simulink model "EV_basic_8_1_triple"  (R2018b)
settings: Solver=VariableStepAuto  StartTime=0.0  StopTime=440  MaxStep=1e-2  MinStep=1e-5  RelTol=1e-2
values from neighbouring files (symbols this model uses):
  Av = 2.75    [InitiateModel.m]    (also in InitiateModel_layouts.m; nurburg_lap.mat)
  batt_max_v = cell_series*cell_max_v    [InitiateModel.m]    (also in nurburg_lap.mat = 613.2)
  Capacity = batt_cap*1e3*3600    (= 252000000)    [InitiateModel.m]    (also in InitiateModel_layouts.m = 252000; nurburg_lap.mat = 180000000)
  Cd = 0.26    [InitiateModel.m]    (also in InitiateModel_layouts.m; nurburg_lap.mat)
  Cr = 0.01    [InitiateModel.m]    (also in InitiateModel_layouts.m; nurburg_lap.mat)
  eta_DC = .985    (= 0.985)    [InitiateModel.m]    (also in InitiateModel_layouts.m; nurburg_lap.mat)
  eta_inv = .965    (= 0.965)    [InitiateModel.m]    (also in InitiateModel_layouts.m; nurburg_lap.mat)
  front_motor = 2    [InitiateModel.m]    (also in nurburg_lap.mat = 0)
  Fv_max = 2*Fv_max_electric    (= 22377.6223776)    [InitiateModel.m]    (also in InitiateModel_layouts.m = 16783.2167832; nurburg_lap.mat)
  Fz_tire = (Mv * weight_dist * 0.5)*9.81    [InitiateModel.m]    (also in nurburg_lap.mat = 5290.7414625)
  gratio = 7    [InitiateModel.m]    (also in InitiateModel_layouts.m = 5.3; nurburg_lap.mat = 5.5)
  grav = 9.81    [InitiateModel.m]    (also in InitiateModel_layouts.m; nurburg_lap.mat)
  inv_eff = 0.98    [InitiateModel.m]    (also in nurburg_lap.mat)
  Ke = 0.607    [InitiateModel.m]    (also in InitiateModel_layouts.m; nurburg_lap.mat)
  max_curr = cell_max_curr*cells_parallel    [InitiateModel.m]    (also in InitiateModel_layouts.m = 270; nurburg_lap.mat = 400)
  motoreff_T = linspace(0,300,101)    [InitiateModel.m]    (also in motoreff_w.mat = [0 4 8 12 16 20 24 28 32 36 40 44 ... (101 elements, 1x101)]; nurburg_lap.mat = [0 3 6 9 12 15 18 21 24 27 30 33 ... (101 elements, 1x101)])
  motoreff_w = [0 18 36 54 72 90 108 126 144 162 180 198 ... (101 elements, 1x101)]    [motoreff_w.mat]    (also in nurburg_lap.mat = [0 12 24 36 48 60 72 84 96 108 120 132 ... (101 elements, 1x)
  Mv = 1420    [InitiateModel.m]    (also in InitiateModel_layouts.m; nurburg_lap.mat)
  opt_slip = 0.18    [InitiateModel.m]    (also in nurburg_lap.mat)
  Pe_max = 160e3    (= 160000)    [InitiateModel.m]    (also in InitiateModel_layouts.m = 120000; nurburg_lap.mat)
  rear_motor = 2    [InitiateModel.m]    (also in nurburg_lap.mat)
  regen_eff = 0.8    [InitiateModel.m]    (also in nurburg_lap.mat)
  rho_air = 1.204    [InitiateModel.m]    (also in InitiateModel_layouts.m; nurburg_lap.mat)
  rw = 0.668/2    (= 0.334)    [InitiateModel.m]    (also in InitiateModel_layouts.m; nurburg_lap.mat)
  s_time = 0.01    [InitiateModel.m]    (also in InitiateModel_layouts.m; nurburg_lap.mat)
  SOC_0 = 80    [InitiateModel.m]    (also in InitiateModel_layouts.m; nurburg_lap.mat)
  Te_max = 2*Te_max_electric    (= 2442.52479547)    [InitiateModel.m]    (also in InitiateModel_layouts.m = 1831.8935966; nurburg_lap.mat)
  tstep = .01    (= 0.01)    [InitiateModel.m]    (also in InitiateModel_layouts.m; nurburg_lap.mat)
  Vbase = 14.30    (= 14.3)    [InitiateModel.m]    (also in InitiateModel_layouts.m; nurburg_lap.mat)
  Vbus_ref = 600    [InitiateModel.m]    (also in InitiateModel_layouts.m = 530; nurburg_lap.mat)
  W_d = 0.5    [InitiateModel.m]    (also in InitiateModel_layouts.m; nurburg_lap.mat)
undefined symbols (not defined in the file or in its folder): MException, throw
libraries: simulink x6, autolibshared x3, autolibdcdc x1
(part 4 of 4)

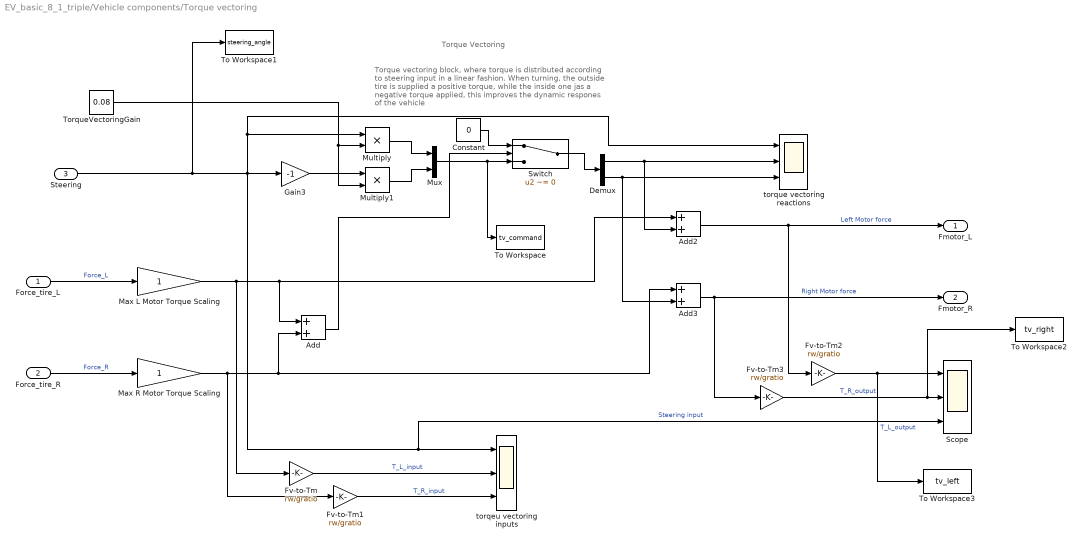
== system EV_basic_8_1_triple/Vehicle components/Torque vectoring ==
  note: Torque vectoring block, where torque is distributed according to steering input in a linear fashion.
      | When turning, the outside tire is supplied a positive torque, while the inside one jas a negative torque applied, this improves the dynamic respones of the vehicle
  note: Torque Vectoring
  Force_tire_L : Inport
  Force_tire_R : Inport  Port=2
  Steering : Inport  Port=3
  Add : Sum
  Add2 : Sum
  Add3 : Sum
  Constant : Constant  Value=0
  Demux : Demux  Outputs=2
  Fv-to-Tm{,1..3} (4 alike) : Gain  Gain=rw/gratio
  Gain3 : Gain  Gain=-1
  Max L Motor Torque Scaling : Gain
  Max R Motor Torque Scaling : Gain
  Multiply : Product  Inputs=**
  Multiply1 : Product  Inputs=**
  Mux : Mux  Inputs=2
  Scope : Scope  NumInputPorts=3
  Switch : Switch  Criteria=u2 ~= 0  Threshold=0.05  ZeroCross=off
  To Workspace : ToWorkspace  VariableName=tv_command  SaveFormat=Structure With Time  SampleTime=-1
  To Workspace1 : ToWorkspace  VariableName=steering_angle  SaveFormat=Structure With Time  SampleTime=-1
  To Workspace2 : ToWorkspace  VariableName=tv_right  SaveFormat=Structure With Time  SampleTime=s_time
  To Workspace3 : ToWorkspace  VariableName=tv_left  SaveFormat=Structure With Time  SampleTime=s_time
  TorqueVectoringGain : Constant  Value=0.08
  torqeu vectoring inputs : Scope  NumInputPorts=3
  torque vectoring reactions : Scope  NumInputPorts=3
  Fmotor_L : Outport
  Fmotor_R : Outport  Port=2
  wires:
  Demux/1 -> Add2/2, torque vectoring reactions/2
  Multiply/1 -> Mux/1
  TorqueVectoringGain/1 -> Multiply1/2, Multiply/2
  Multiply1/1 -> Mux/2
  Add/1 -> Switch/2
  Force_tire_L/1 -> Max L Motor Torque Scaling/1  "Force_L"
  Steering/1 -> To Workspace1/1, Multiply/1, torque vectoring reactions/1, Scope/3, torqeu vectoring inputs/1, Gain3/1  "Steering input"
  Add2/1 -> Fv-to-Tm2/1, Fmotor_L/1  "Left Motor force"
  Gain3/1 -> Multiply1/1
  Max L Motor Torque Scaling/1 -> Fv-to-Tm/1, Add/1, Add2/1
  Constant/1 -> Switch/1
  Switch/1 -> Demux/1
  Mux/1 -> To Workspace/1, Switch/3
  Add3/1 -> Fv-to-Tm3/1, Fmotor_R/1  "Right Motor force"
  Max R Motor Torque Scaling/1 -> Fv-to-Tm1/1, Add/2, Add3/1
  Force_tire_R/1 -> Max R Motor Torque Scaling/1  "Force_R"
  Fv-to-Tm1/1 -> torqeu vectoring inputs/3  "T_R_input"
  Fv-to-Tm/1 -> torqeu vectoring inputs/2  "T_L_input"
  Demux/2 -> torque vectoring reactions/3, Add3/2
  Fv-to-Tm2/1 -> To Workspace3/1, Scope/1  "T_L_output"
  Fv-to-Tm3/1 -> To Workspace2/1, Scope/2  "T_R_output"

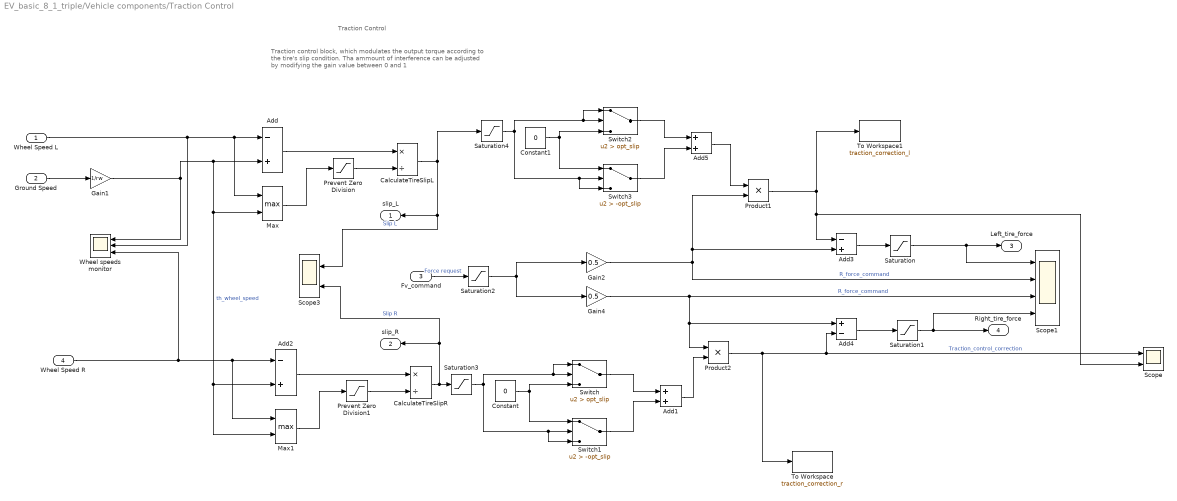
== system EV_basic_8_1_triple/Vehicle components/Traction Control ==
  note: Traction control block, which modulates the output torque according to the tire's slip condition. Tha ammount of interference can be adjusted by modifying the gain value between 0 and 1
  note: Traction Control
  Wheel Speed L : Inport
  Ground Speed : Inport  Port=2
  Fv_command : Inport  Port=3
  Wheel Speed R : Inport  Port=4
  Add : Sum  Inputs=-+
  Add1 : Sum
  Add2 : Sum  Inputs=-+
  Add3 : Sum  Inputs=-+
  Add4 : Sum  Inputs=+-
  Add5 : Sum
  CalculateTireSlipL : Product  Inputs=*/
  CalculateTireSlipR : Product  Inputs=*/
  Constant : Constant  Value=0
  Constant1 : Constant  Value=0
  Gain1 : Gain  Gain=1/rw
  Gain2 : Gain  Gain=0.5
  Gain4 : Gain  Gain=0.5
  Max : MinMax  Function=max  Inputs=2
  Max1 : MinMax  Function=max  Inputs=2
  Prevent Zero Division : Saturate  UpperLimit=1000  LowerLimit=0.0001
  Prevent Zero Division1 : Saturate  UpperLimit=1000  LowerLimit=0.0001
  Product1 : Product
  Product2 : Product
  Saturation : Saturate  UpperLimit=Te_max*(0.5*front_motor+0.5*rear_motor)*(gratio/rw)*0.5  LowerLimit=-Te_max*(0.5*front_motor+0.5*rear_motor)*(gratio/rw)*0.5
  Saturation1 : Saturate  UpperLimit=Te_max*(0.5*front_motor+0.5*rear_motor)*(gratio/rw)*0.5  LowerLimit=-Te_max*(0.5*front_motor+0.5*rear_motor)*(gratio/rw)*0.5
  Saturation2 : Saturate  UpperLimit=Te_max*(0.5*front_motor+0.5*rear_motor)*(gratio/rw)  LowerLimit=-Te_max*(0.5*front_motor+0.5*rear_motor)*(gratio/rw)
  Saturation3 : Saturate  UpperLimit=0.8  LowerLimit=-0.8
  Saturation4 : Saturate  UpperLimit=0.8  LowerLimit=-0.8
  Scope : Scope  NumInputPorts=2
  Scope1 : Scope  NumInputPorts=4
  Scope3 : Scope  NumInputPorts=2
  Switch : Switch  Criteria=u2 > Threshold  Threshold=opt_slip  ZeroCross=off
  Switch1 : Switch  Criteria=u2 > Threshold  Threshold=-opt_slip  ZeroCross=off
  Switch2 : Switch  Criteria=u2 > Threshold  Threshold=opt_slip  ZeroCross=off
  Switch3 : Switch  Criteria=u2 > Threshold  Threshold=-opt_slip  ZeroCross=off
  To Workspace : ToWorkspace  VariableName=traction_correction_r  SaveFormat=Structure With Time  SampleTime=s_time
  To Workspace1 : ToWorkspace  VariableName=traction_correction_l  SaveFormat=Structure With Time  SampleTime=s_time
  Wheel speeds monitor : Scope  NumInputPorts=3
  slip_L : Outport
  slip_R : Outport  Port=2
  Left_tire_force : Outport  Port=3
  Right_tire_force : Outport  Port=4
  wires:
  Prevent Zero Division/1 -> CalculateTireSlipL/2
  Max/1 -> Prevent Zero Division/1
  Wheel Speed L/1 -> Wheel speeds monitor/2, Max/1, Add/1
  Add/1 -> CalculateTireSlipL/1
  Wheel Speed R/1 -> Wheel speeds monitor/3, Max1/1, Add2/1
  Max1/1 -> Prevent Zero Division1/1
  Prevent Zero Division1/1 -> CalculateTireSlipR/2
  Ground Speed/1 -> Gain1/1
  Add2/1 -> CalculateTireSlipR/1
  Gain1/1 -> Max/2, Max1/2, Add2/2, Add/2, Wheel speeds monitor/1  "th_wheel_speed"
  Gain4/1 -> Product2/1, Add4/1, Scope1/3  "R_force_command"
  Fv_command/1 -> Saturation2/1  "Force request"
  Gain2/1 -> Add3/2, Product1/2, Scope1/2  "R_force_command"
  Saturation/1 -> Scope1/1, Left_tire_force/1
  Saturation1/1 -> Right_tire_force/1, Scope1/4
  Add3/1 -> Saturation/1
  Product2/1 -> To Workspace/1, Scope/1, Add4/2  "Traction_control_correction"
  CalculateTireSlipR/1 -> Scope3/2, slip_R/1, Saturation3/1  "Slip R"
  Add4/1 -> Saturation1/1
  Saturation2/1 -> Gain2/1, Gain4/1
  CalculateTireSlipL/1 -> Saturation4/1, Scope3/1, slip_L/1  "Slip L"
  Product1/1 -> To Workspace1/1, Scope/2, Add3/1
  Constant/1 -> Switch1/1, Switch/3
  Switch1/1 -> Add1/2
  Switch/1 -> Add1/1
  Add1/1 -> Product2/2
  Saturation3/1 -> Switch1/3, Switch1/2, Switch/1, Switch/2
  Switch2/1 -> Add5/1
  Saturation4/1 -> Switch3/3, Switch3/2, Switch2/1, Switch2/2
  Switch3/1 -> Add5/2
  Constant1/1 -> Switch3/1, Switch2/3
  Add5/1 -> Product1/1

== system EV_basic_8_1_triple/Vehicle components/Left Drive Inverter: Functional/Inverter Controller ==
  note: Inverter is kept in phase with rotor, and torque command is used
      | to directly set peak currents, which ultimately determine engine torque.
      | Because ideal sensing/control are assumed, no dynamics are considered
  note: Inverter Functional Controller
  Tactual : Inport
  thetar : Inport  Port=2
  Saturation : Saturate  UpperLimit=500  LowerLimit=-500
  Torque [Nm] to Inverter Peak Current [A] : Gain  Gain=1/Ke*2/3
  Ipk : Outport
  thetai : Outport  Port=2
  wires:
  thetar/1 -> thetai/1
  Torque [Nm] to Inverter Peak Current [A]/1 -> Saturation/1
  Tactual/1 -> Torque [Nm] to Inverter Peak Current [A]/1
  Saturation/1 -> Ipk/1

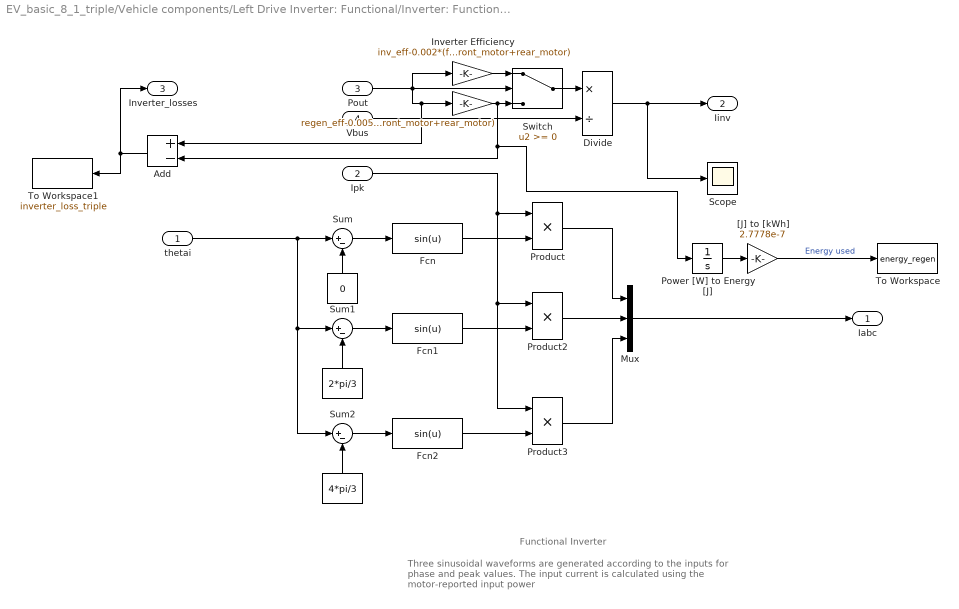
== system EV_basic_8_1_triple/Vehicle components/Left Drive Inverter: Functional/Inverter: Functional ==
  note: Three sinusoidal waveforms are generated according to the inputs
      | for phase and peak values.  The input current is calculated using
      | the motor-reported input power
  note: Functional Inverter
  thetai : Inport
  Ipk : Inport  Port=2
  Pout : Inport  Port=3
  Vbus : Inport  Port=4
  " " : Gain  Gain=regen_eff-0.005*(front_motor+rear_motor)
  " " : Constant  Value=0
  "   " : Constant  Value=2*pi/3
  "    " : Constant  Value=4*pi/3
  " Fcn" : Fcn  Expr=sin(u)
  Add : Sum  Inputs=+-
  Divide : Product  Inputs=*/
  Fcn1 : Fcn  Expr=sin(u)
  Fcn2 : Fcn  Expr=sin(u)
  Inverter Efficiency : Gain  Gain=inv_eff-0.002*(front_motor+rear_motor)
  Mux : Mux  Inputs=3
  Power [W] to Energy [J] : Integrator
  Product : Product  RndMeth=Zero
  Product2 : Product  RndMeth=Zero
  Product3 : Product  RndMeth=Zero
  Scope : Scope
  Sum : Sum  Inputs=|+-
  Sum1 : Sum  Inputs=|+-
  Sum2 : Sum  Inputs=|+-
  Switch : Switch
  To Workspace : ToWorkspace  VariableName=energy_regen  SaveFormat=Structure With Time  SampleTime=s_time
  To Workspace1 : ToWorkspace  VariableName=inverter_loss_triple  SaveFormat=Timeseries  SampleTime=-1
  "[J] to [kWh]" : Gain  Gain=2.7778e-7
  Iabc : Outport
  Iinv : Outport  Port=2
  Inverter_losses : Outport  Port=3
  wires:
  " Fcn"/1 -> Product/2
  Product/1 -> Mux/1
  Ipk/1 -> Product/1, Product2/1, Product3/1
  Sum/1 -> " Fcn"/1
  Fcn1/1 -> Product2/2
  Sum1/1 -> Fcn1/1
  Fcn2/1 -> Product3/2
  Sum2/1 -> Fcn2/1
  Product2/1 -> Mux/2
  Product3/1 -> Mux/3
  " "/1 -> Sum/2
  "   "/1 -> Sum1/2
  "    "/1 -> Sum2/2
  thetai/1 -> Sum/1, Sum1/1, Sum2/1
  Mux/1 -> Iabc/1
  Pout/1 -> Switch/2, Inverter Efficiency/1, Add/1, " "/1
  Vbus/1 -> Divide/2
  Divide/1 -> Scope/1, Iinv/1
  Switch/1 -> Divide/1
  Inverter Efficiency/1 -> Switch/1
  " "/1 -> Add/2, Power [W] to Energy [J]/1, Switch/3
  "[J] to [kWh]"/1 -> To Workspace/1  "Energy used"
  Power [W] to Energy [J]/1 -> "[J] to [kWh]"/1
  Add/1 -> To Workspace1/1, Inverter_losses/1

== system EV_basic_8_1_triple/Vehicle components/Left Drive Inverter: Functional/Motor Limits Model ==
  note: Electric Motor Limits Model
  note: Model enforces power and torque limits of engine
  wr : Inport
  Tmcommand : Inport  Port=2
  Engine Max Power : Saturate  UpperLimit=Pe_max*0.5*(0.5*front_motor+0.5*rear_motor)  LowerLimit=-Pe_max*0.5*(0.5*front_motor+0.5*rear_motor)
  Engine Max Torque : Saturate  UpperLimit=Te_max*1.3  LowerLimit=-Te_max*1.3
  Engine Max Torque1 : Saturate  UpperLimit=Te_max*0.5*(0.5*front_motor+0.5*rear_motor)  LowerLimit=-Te_max*0.5*(0.5*front_motor+0.5*rear_motor)
  Gearing Reduction : Gain  Gain=1/gratio
  Memory : Memory
  P=Tw : Product  RndMeth=Zero
  Scope : Scope  NumInputPorts=2
  Switch : Switch  Criteria=u2 ~= 0
  T=P/w : Product  Inputs=*/
  Torque or Power Limited Operation : simulink/Logic and Bit Operations/Compare To Constant  relop=<  const=Vbase  OutDataTypeStr=uint8  ZeroCross=off
  angular [rad/s]  to Linear [m/s] : Gain  Gain=rw
  Tactual : Outport
  wires:
  P=Tw/1 -> Engine Max Power/1  "Pm"
  Engine Max Power/1 -> T=P/w/1  "Pactual"
  Switch/1 -> Memory/1
  T=P/w/1 -> Engine Max Torque/1
  Torque or Power Limited Operation/1 -> Scope/1, Switch/2
  Memory/1 -> Tactual/1
  angular [rad/s]  to Linear [m/s]/1 -> Gearing Reduction/1
  wr/1 -> P=Tw/2, T=P/w/2, Scope/2, angular [rad/s]  to Linear [m/s]/1  "Rotor Angular Speed"
  Gearing Reduction/1 -> Torque or Power Limited Operation/1
  Engine Max Torque1/1 -> Switch/1
  Engine Max Torque/1 -> Switch/3
  Tmcommand/1 -> Engine Max Torque1/1, P=Tw/1

== system EV_basic_8_1_triple/Vehicle components/PMAC Motor Left: Functional/Ideal Motor Model ==
  note: Electric torque for PMAC is determined according to the three
      | current phases and their relative position to the rotor.
  note: PMAC Ideal Motor Electronic Torque Model
  Ia : Inport
  Ib : Inport  Port=2
  Ic : Inport  Port=3
  pihr : Inport  Port=4
  Add : Sum  Inputs=+++
  Angle between rotor and pole a : Fcn  Expr=sin(u)
  Angle between rotor and pole b : Fcn  Expr=sin(u-2*pi/3)
  Angle between rotor and pole c : Fcn  Expr=sin(u-4*pi/3)
  Product : Product  RndMeth=Zero
  Product1 : Product  RndMeth=Zero
  Product2 : Product  RndMeth=Zero
  Torque Constant : Gain  Gain=Ke
  Tm : Outport
  wires:
  pihr/1 -> Angle between rotor and pole a/1, Angle between rotor and pole b/1, Angle between rotor and pole c/1
  Angle between rotor and pole a/1 -> Product/2
  Ia/1 -> Product/1
  Ib/1 -> Product1/1
  Angle between rotor and pole b/1 -> Product1/2
  Ic/1 -> Product2/1
  Angle between rotor and pole c/1 -> Product2/2
  Add/1 -> Torque Constant/1
  Product/1 -> Add/1
  Product1/1 -> Add/2
  Product2/1 -> Add/3
  Torque Constant/1 -> Tm/1

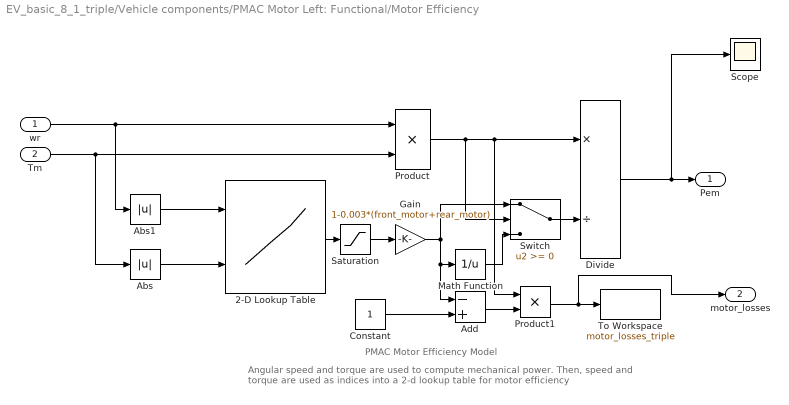
== system EV_basic_8_1_triple/Vehicle components/PMAC Motor Left: Functional/Motor Efficiency ==
  note: PMAC Motor Efficiency Model
  note: Angular speed and torque are used to compute mechanical power.  Then, speed
      | and torque are used as indices into a 2-d lookup table for motor efficiency
  wr : Inport
  Tm : Inport  Port=2
  2-D Lookup Table : Lookup_n-D  BreakpointsForDimension1=motoreff_w  BreakpointsForDimension2=motoreff_T  BeginIndexSearchUsingPreviousIndexResult=on  Table=motoreff'  UseLastTableValue=on  RndMeth=Simplest  InputSameDT=on
  Abs : Abs
  Abs1 : Abs
  Add : Sum  Inputs=-+
  Constant : Constant
  Divide : Product  Inputs=*/
  Gain : Gain  Gain=1-0.003*(front_motor+rear_motor)
  Math Function : Math  Operator=reciprocal  SaturateOnIntegerOverflow=on
  Product : Product  RndMeth=Zero
  Product1 : Product
  Saturation : Saturate  UpperLimit=1  LowerLimit=.3
  Scope : Scope
  Switch : Switch
  To Workspace : ToWorkspace  VariableName=motor_losses_triple  SaveFormat=Structure With Time  SampleTime=s_time
  Pem : Outport
  motor_losses : Outport  Port=2
  wires:
  Divide/1 -> Scope/1, Pem/1
  Abs/1 -> 2-D Lookup Table/2
  Abs1/1 -> 2-D Lookup Table/1
  2-D Lookup Table/1 -> Saturation/1
  wr/1 -> Abs1/1, Product/1
  Tm/1 -> Abs/1, Product/2
  Switch/1 -> Divide/2
  Product/1 -> Product1/1, Divide/1, Switch/2
  Saturation/1 -> Gain/1
  Math Function/1 -> Switch/3
  Constant/1 -> Add/2
  Add/1 -> Product1/2
  Product1/1 -> motor_losses/1, To Workspace/1
  Gain/1 -> Add/1, Math Function/1, Switch/1

== system EV_basic_8_1_triple/Vehicle components/PMAC Motor Right: Functional/Ideal Motor Model ==
  note: Electric torque for PMAC is determined according to the three
      | current phases and their relative position to the rotor.
  note: PMAC Ideal Motor Electronic Torque Model
  Ia : Inport
  Ib : Inport  Port=2
  Ic : Inport  Port=3
  pihr : Inport  Port=4
  Add : Sum  Inputs=+++
  Angle between rotor and pole a : Fcn  Expr=sin(u)
  Angle between rotor and pole b : Fcn  Expr=sin(u-2*pi/3)
  Angle between rotor and pole c : Fcn  Expr=sin(u-4*pi/3)
  Product : Product  RndMeth=Zero
  Product1 : Product  RndMeth=Zero
  Product2 : Product  RndMeth=Zero
  Torque Constant : Gain  Gain=Ke
  Tm : Outport
  wires:
  pihr/1 -> Angle between rotor and pole a/1, Angle between rotor and pole b/1, Angle between rotor and pole c/1
  Angle between rotor and pole a/1 -> Product/2
  Ia/1 -> Product/1
  Ib/1 -> Product1/1
  Angle between rotor and pole b/1 -> Product1/2
  Ic/1 -> Product2/1
  Angle between rotor and pole c/1 -> Product2/2
  Add/1 -> Torque Constant/1
  Product/1 -> Add/1
  Product1/1 -> Add/2
  Product2/1 -> Add/3
  Torque Constant/1 -> Tm/1

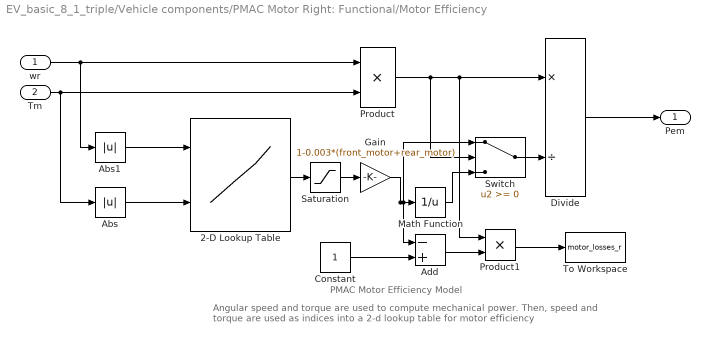
== system EV_basic_8_1_triple/Vehicle components/PMAC Motor Right: Functional/Motor Efficiency ==
  note: PMAC Motor Efficiency Model
  note: Angular speed and torque are used to compute mechanical power.  Then, speed
      | and torque are used as indices into a 2-d lookup table for motor efficiency
  wr : Inport
  Tm : Inport  Port=2
  2-D Lookup Table : Lookup_n-D  BreakpointsForDimension1=motoreff_w  BreakpointsForDimension2=motoreff_T  BeginIndexSearchUsingPreviousIndexResult=on  Table=motoreff'  UseLastTableValue=on  RndMeth=Simplest  InputSameDT=on
  Abs : Abs
  Abs1 : Abs
  Add : Sum  Inputs=-+
  Constant : Constant
  Divide : Product  Inputs=*/
  Gain : Gain  Gain=1-0.003*(front_motor+rear_motor)
  Math Function : Math  Operator=reciprocal  SaturateOnIntegerOverflow=on
  Product : Product  RndMeth=Zero
  Product1 : Product
  Saturation : Saturate  UpperLimit=1  LowerLimit=.05
  Switch : Switch
  To Workspace : ToWorkspace  VariableName=motor_losses_r  SaveFormat=Structure With Time  SampleTime=s_time
  Pem : Outport
  wires:
  Divide/1 -> Pem/1
  Abs/1 -> 2-D Lookup Table/2
  Abs1/1 -> 2-D Lookup Table/1
  2-D Lookup Table/1 -> Saturation/1
  wr/1 -> Abs1/1, Product/1
  Tm/1 -> Abs/1, Product/2
  Switch/1 -> Divide/2
  Math Function/1 -> Switch/3
  Constant/1 -> Add/2
  Product1/1 -> To Workspace/1
  Add/1 -> Product1/2
  Saturation/1 -> Gain/1
  Product/1 -> Product1/1, Divide/1, Switch/2
  Gain/1 -> Add/1, Switch/1, Math Function/1

== system EV_basic_8_1_triple/Vehicle components/Right Drive Inverter: Functional/Inverter Controller ==
  note: Inverter is kept in phase with rotor, and torque command is used
      | to directly set peak currents, which ultimately determine engine torque.
      | Because ideal sensing/control are assumed, no dynamics are considered
  note: Inverter Functional Controller
  Tactual : Inport
  thetar : Inport  Port=2
  Saturation : Saturate  UpperLimit=500  LowerLimit=-500
  Torque [Nm] to Inverter Peak Current [A] : Gain  Gain=1/Ke*2/3
  Ipk : Outport
  thetai : Outport  Port=2
  wires:
  thetar/1 -> thetai/1
  Torque [Nm] to Inverter Peak Current [A]/1 -> Saturation/1
  Tactual/1 -> Torque [Nm] to Inverter Peak Current [A]/1
  Saturation/1 -> Ipk/1

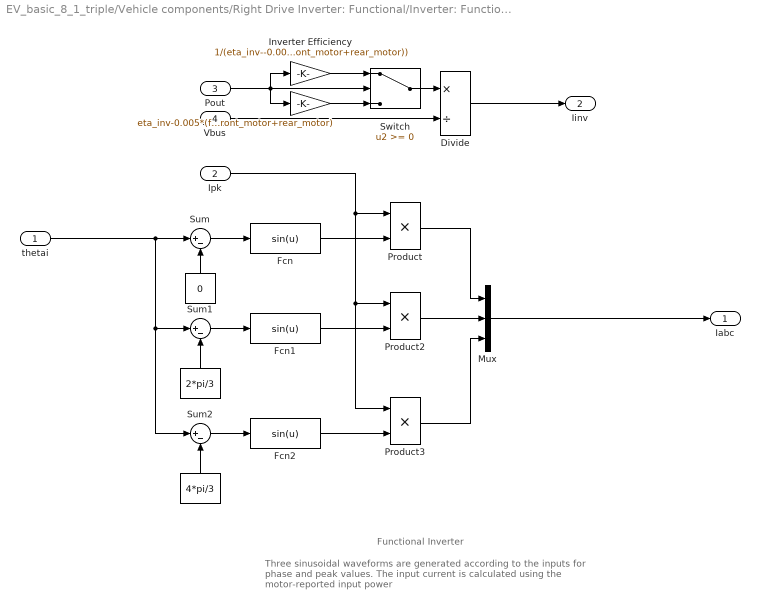
== system EV_basic_8_1_triple/Vehicle components/Right Drive Inverter: Functional/Inverter: Functional ==
  note: Three sinusoidal waveforms are generated according to the inputs
      | for phase and peak values.  The input current is calculated using
      | the motor-reported input power
  note: Functional Inverter
  thetai : Inport
  Ipk : Inport  Port=2
  Pout : Inport  Port=3
  Vbus : Inport  Port=4
  " " : Gain  Gain=eta_inv-0.005*(front_motor+rear_motor)
  " " : Constant  Value=0
  "   " : Constant  Value=2*pi/3
  "    " : Constant  Value=4*pi/3
  " Fcn" : Fcn  Expr=sin(u)
  Divide : Product  Inputs=*/
  Fcn1 : Fcn  Expr=sin(u)
  Fcn2 : Fcn  Expr=sin(u)
  Inverter Efficiency : Gain  Gain=1/(eta_inv--0.005*(front_motor+rear_motor))
  Mux : Mux  Inputs=3
  Product : Product  RndMeth=Zero
  Product2 : Product  RndMeth=Zero
  Product3 : Product  RndMeth=Zero
  Sum : Sum  Inputs=|+-
  Sum1 : Sum  Inputs=|+-
  Sum2 : Sum  Inputs=|+-
  Switch : Switch
  Iabc : Outport
  Iinv : Outport  Port=2
  wires:
  " Fcn"/1 -> Product/2
  Product/1 -> Mux/1
  Ipk/1 -> Product/1, Product2/1, Product3/1
  Sum/1 -> " Fcn"/1
  Fcn1/1 -> Product2/2
  Sum1/1 -> Fcn1/1
  Fcn2/1 -> Product3/2
  Sum2/1 -> Fcn2/1
  Product2/1 -> Mux/2
  Product3/1 -> Mux/3
  " "/1 -> Sum/2
  "   "/1 -> Sum1/2
  "    "/1 -> Sum2/2
  thetai/1 -> Sum/1, Sum1/1, Sum2/1
  Mux/1 -> Iabc/1
  Pout/1 -> Switch/2, Inverter Efficiency/1, " "/1
  Vbus/1 -> Divide/2
  Divide/1 -> Iinv/1
  Switch/1 -> Divide/1
  Inverter Efficiency/1 -> Switch/1
  " "/1 -> Switch/3

== system EV_basic_8_1_triple/Vehicle components/Right Drive Inverter: Functional/Motor Limits Model ==
  note: Electric Motor Limits Model
  note: Model enforces power and torque limits of engine
  wr : Inport
  Tmcommand : Inport  Port=2
  Engine Max Power : Saturate  UpperLimit=Pe_max*0.5*(0.5*front_motor+0.5*rear_motor)  LowerLimit=-Pe_max*0.5*(0.5*front_motor+0.5*rear_motor)
  Engine Max Torque : Saturate  UpperLimit=Te_max*0.5*(0.5*front_motor+0.5*rear_motor)  LowerLimit=-Te_max*0.5*(0.5*front_motor+0.5*rear_motor)
  Engine Max Torque1 : Saturate  UpperLimit=Te_max*1.3  LowerLimit=-Te_max*1.3
  Gearing Reduction : Gain  Gain=1/gratio
  Memory : Memory
  P=Tw : Product  RndMeth=Zero
  Switch : Switch  Criteria=u2 ~= 0
  T=P/w : Product  Inputs=*/
  Torque or Power Limited Operation : simulink/Logic and Bit Operations/Compare To Constant  relop=<  const=Vbase  OutDataTypeStr=uint8  ZeroCross=off
  angular [rad/s]  to Linear [m/s] : Gain  Gain=rw
  Tactual : Outport
  wires:
  Tmcommand/1 -> P=Tw/1, Engine Max Torque/1
  P=Tw/1 -> Engine Max Power/1  "Pm"
  Engine Max Power/1 -> T=P/w/1  "Pactual"
  Switch/1 -> Memory/1
  T=P/w/1 -> Engine Max Torque1/1
  Torque or Power Limited Operation/1 -> Switch/2
  Engine Max Torque/1 -> Switch/1
  Memory/1 -> Tactual/1
  angular [rad/s]  to Linear [m/s]/1 -> Gearing Reduction/1
  wr/1 -> P=Tw/2, T=P/w/2, angular [rad/s]  to Linear [m/s]/1  "Rotor Angular Speed"
  Gearing Reduction/1 -> Torque or Power Limited Operation/1
  Engine Max Torque1/1 -> Switch/3

== system EV_basic_8_1_triple/Vehicle components/Subsystem/DC-DC Converter: Functional ==
  note: DC-DC converter consists of power stage
      | model and controller, which drives the bus
      | voltage to a given reference by varying
      | converter duty cycle
  note: DC-DC Functional Model
  Vref : Inport
  Vbat : Inport  Port=2
  Iout : Inport  Port=3
  Battery current limiter for protection : Saturate  Commented=through  UpperLimit=max_curr*1.2  LowerLimit=max_curr
  DC/DC Controller1 : Subsystem
  "DC/DC Model: Functional " : Subsystem
  Vbus : Outport
  Ibat : Outport  Port=2
  wires:
  "DC/DC Model: Functional "/1(Vout) -> DC/DC Controller1/1(Vbus), Vbus/1
  DC/DC Controller1/1(D) -> "DC/DC Model: Functional "/3(D)
  Vref/1 -> DC/DC Controller1/2(Vref)
  Iout/1 -> Battery current limiter for protection/1
  Vbat/1 -> "DC/DC Model: Functional "/2(Vbat)
  "DC/DC Model: Functional "/2(Ibat) -> Ibat/1
  Battery current limiter for protection/1 -> "DC/DC Model: Functional "/1(Iout)

== system EV_basic_8_1_triple/Vehicle components/Subsystem/DC-DC Converter: Functional/DC//DC Controller1 ==
  note: Basic PWM controller for DC-DC Boost converter.
      | Compensator is pure integral to ensure zero
      | steady-state error.  No dynamics considered. Duty
      | cycle is limited between 0 and 1
  note: DC-DC Functional Controller
  Vbus : Inport
  Vref : Inport  Port=2
  Gain : Gain
  Integrator : Integrator  InitialCondition=.5
  Saturation : Saturate  UpperLimit=1  LowerLimit=0
  Sum : Sum  Inputs=|-+
  D : Outport
  wires:
  Gain/1 -> Integrator/1
  Integrator/1 -> Saturation/1
  Sum/1 -> Gain/1
  Vbus/1 -> Sum/1
  Vref/1 -> Sum/2
  Saturation/1 -> D/1

== system EV_basic_8_1_triple/Vehicle components/Subsystem/DC-DC Converter: Functional/DC//DC Model: Functional  ==
  note: Functional Mmodel of lossless DC-DC Converter.
      | Boost converter is assumed, and ideal conversion
      | ratio is used
  note: DC-DC Functional Model
  Iout : Inport
  Vbat : Inport  Port=2
  D : Inport  Port=3
  " " : Gain  Gain=eta_DC
  Add : Sum  Inputs=+-
  Constant : Constant
  Converter Efficiency : Gain  Gain=eta_DC
  Divide : Product  Inputs=*/
  Divide1 : Product  Inputs=/*
  Scope : Scope
  Switch : Switch
  Vout : Outport
  Ibat : Outport  Port=2
  wires:
  Constant/1 -> Add/1
  D/1 -> Add/2
  Add/1 -> Divide/2, Divide1/1  "Dprime"
  Vbat/1 -> Divide/1
  Divide/1 -> Vout/1
  Iout/1 -> Scope/1, Switch/2, Converter Efficiency/1, " "/1
  Divide1/1 -> Ibat/1
  Switch/1 -> Divide1/2
  Converter Efficiency/1 -> Switch/1
  " "/1 -> Switch/3
